simulink model "DR_Aufgabe02"  (R2022a)
settings: Solver=FixedStepAuto  StartTime=0.0  StopTime=10  FixedStep=0.0005  RelTol=1e-3
values from neighbouring files (symbols this model uses):
  den_F_d = [1, d1_d]    [Aufgabe02_Parameter.m]
  J = 4.2e-4    (= 0.00042)    [Aufgabe02_Parameter.m]
  Ki_sum_b = Ki_b_impl * T / 2    [Aufgabe02_Parameter.m]
  Ki_sum_d = Ki_d_impl * T / 2    [Aufgabe02_Parameter.m]
  Kp_b_impl = K_DBO_b * (1 + z_N_b) / 2    [Aufgabe02_Parameter.m]
  Kp_d_impl = K_DBO_d * (1 + z_N_d) / 2    [Aufgabe02_Parameter.m]
  M_max = 0.15    [Aufgabe02_Parameter.m]
  num_F_d = [(1 + d1_d), 0]    [Aufgabe02_Parameter.m]
  T_sigma_omega = 0.003    [Aufgabe02_Parameter.m]
settings Model: Creator=Youkun Mao  LastModifiedBy=Youkun Mao
settings ModelReferenceCC: EnableRefExpFcnMdlSchedulingChecks=off
settings RTWCC: Description=Generic Real-Time Target  GPUComputeCapability=5.0

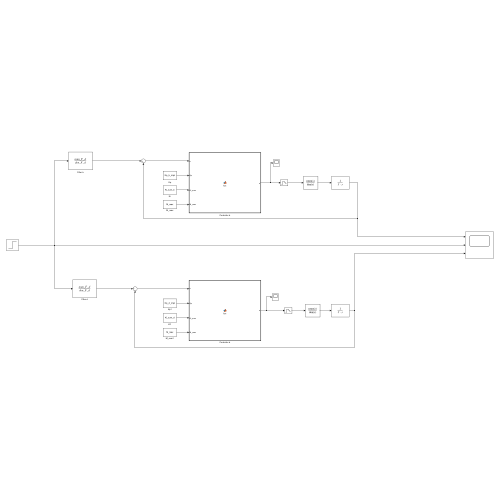
[thumbnail: Simulink's stored preview of the top-level diagram]
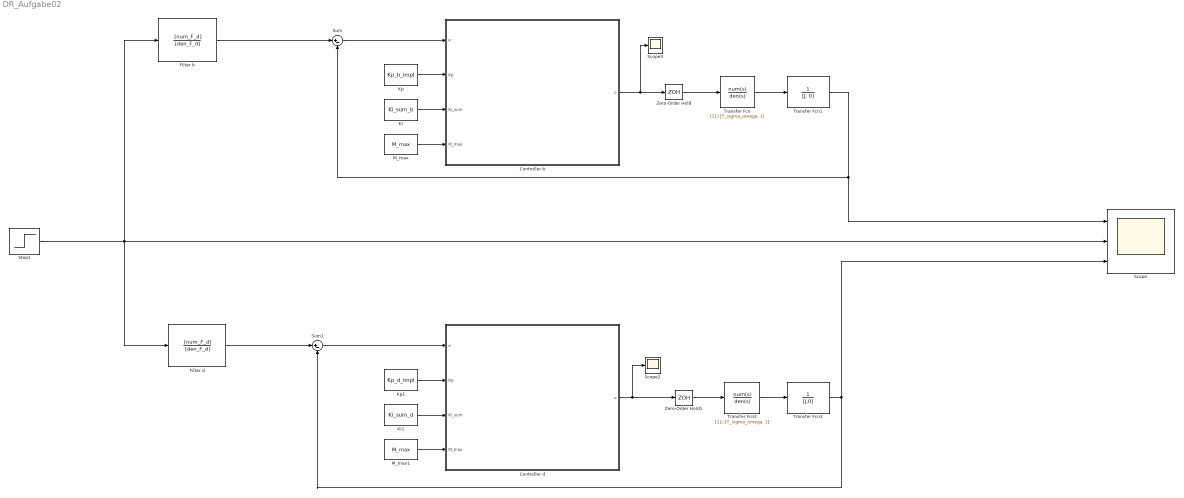
== system DR_Aufgabe02 ==
  Controller b : MATLAB Function  TreatAsAtomicUnit=on
  Controller d : MATLAB Function  TreatAsAtomicUnit=on
  Filter b : DiscreteTransferFcn  Numerator=[num_F_d]  Denominator=[den_F_d]
  Filter d : DiscreteTransferFcn  Numerator=[num_F_d]  Denominator=[den_F_d]
  Ki : Constant  Value=Ki_sum_b
  Ki1 : Constant  Value=Ki_sum_d
  Kp : Constant  Value=Kp_b_impl
  Kp1 : Constant  Value=Kp_d_impl
  M_max : Constant  Value=M_max
  M_max1 : Constant  Value=M_max
  Scope : Scope  NumInputPorts=3
  Scope2 : Scope
  Scope3 : Scope
  Step1 : Step  Time=0.01  After=100  SampleTime=0
  Sum : Sum  Inputs=|+-
  Sum1 : Sum  Inputs=|+-
  Transfer Fcn : TransferFcn  Denominator=[T_sigma_omega, 1]
  Transfer Fcn1 : TransferFcn  Denominator=[J, 0]
  Transfer Fcn2 : TransferFcn  Denominator=[T_sigma_omega, 1]
  Transfer Fcn3 : TransferFcn  Denominator=[J,0]
  Zero-Order Hold : ZeroOrderHold  SampleTime=0.0005
  Zero-Order Hold1 : ZeroOrderHold  SampleTime=0.0005
  wires:
  Step1/1 -> Filter b/1, Scope/2, Filter d/1
  Transfer Fcn1/1 -> Scope/1, Sum/2
  Transfer Fcn/1 -> Transfer Fcn1/1
  Zero-Order Hold/1 -> Transfer Fcn/1
  Controller b/1(u) -> Scope3/1, Zero-Order Hold/1
  Sum/1 -> Controller b/1(e)
  M_max/1 -> Controller b/4(M_max)
  Ki/1 -> Controller b/3(Ki_sum)
  Kp/1 -> Controller b/2(Kp)
  Transfer Fcn2/1 -> Transfer Fcn3/1
  Zero-Order Hold1/1 -> Transfer Fcn2/1
  M_max1/1 -> Controller d/4(M_max)
  Ki1/1 -> Controller d/3(Ki_sum)
  Controller d/1(u) -> Scope2/1, Zero-Order Hold1/1
  Sum1/1 -> Controller d/1(e)
  Kp1/1 -> Controller d/2(Kp)
  Transfer Fcn3/1 -> Scope/3, Sum1/2
  Filter d/1 -> Sum1/1
  Filter b/1 -> Sum/1

== matlab function DR_Aufgabe02/Controller d ==
  settings: updateMethod=DISCRETE
  data: e input; u output; Kp input; Ki_sum input; M_max input
function u = fcn(e, Kp, Ki_sum, M_max)
    % discrete PI Controller with Trapezoidal Rule and ARW
    % e: Error input
    % Kp, Ki_sum: Calculated parameters from init script
    % M_max: Torque limit
    
    % Define persistent variables to store state between steps
    persistent e_prev u_I_prev
    if isempty(e_prev)
        e_prev = 0;
        u_I_prev = 0;
    end
    
    % Calculate P-Part
    u_P = Kp * e;
    
    % Calculate I-Part (Trapezoidal Rule) WITHOUT update yet
    % u_I_new = u_I_old + Ki_sum * (e_k + e_{k-1})
    u_I_temp = u_I_prev + Ki_sum * (e + e_prev);
    
    % Calculate Total Unbounded Output
    u_ges = u_P + u_I_temp;
    
    % Anti-Reset-Windup (ARW) & Output Limiting
    if u_ges > M_max
        u = M_max;
    elseif u_ges < -M_max
        u = -M_max;
    else
        u = u_ges;
        u_I_prev = u_I_temp;
    end
    
    e_prev = e;
end

== matlab function DR_Aufgabe02/Controller b ==
  settings: updateMethod=DISCRETE
  data: e input; u output; Kp input; Ki_sum input; M_max input
function u = fcn(e, Kp, Ki_sum, M_max)
    % discrete PI Controller with Trapezoidal Rule and ARW
    % e: Error input
    % Kp, Ki_sum: Calculated parameters from init script
    % M_max: Torque limit
    
    % Define persistent variables to store state between steps
    persistent e_prev u_I_prev
    if isempty(e_prev)
        e_prev = 0;
        u_I_prev = 0;
    end
    
    % Calculate P-Part
    u_P = Kp * e;
    
    % Calculate I-Part (Trapezoidal Rule) WITHOUT update yet
    % u_I_new = u_I_old + Ki_sum * (e_k + e_{k-1})
    u_I_temp = u_I_prev + Ki_sum * (e + e_prev);
    
    % Calculate Total Unbounded Output
    u_ges = u_P + u_I_temp;
    
    % Anti-Reset-Windup (ARW) & Output Limiting
    if u_ges > M_max
        u = M_max;
    elseif u_ges < -M_max
        u = -M_max;
    else
        u = u_ges;
        u_I_prev = u_I_temp;
    end
    
    e_prev = e;
end
